simulink model "camara_simul"  (R2018a)
settings: Solver=VariableStepAuto  StartTime=0.0  StopTime=inf  RelTol=1e-3
undefined symbols (not defined in the file or in its folder): IsPositionTracked, IsSkeletonTracked, JointDepthIndices, JointImageIndices, JointTrackingState, JointWorldCoordinates, none, PositionDepthIndices, PositionImageIndices, PositionWorldCoordinates, Rec, SDTV, SegmentationData, SkeletonTrackingID, videoinput
libraries: visionsinks x3, visionconversions x2, simulink x2, visionstatistics x1, visiontextngfix x1, imaqlib x1
settings Model: Creator=Luís Miranda  LastModifiedBy=Luís Miranda

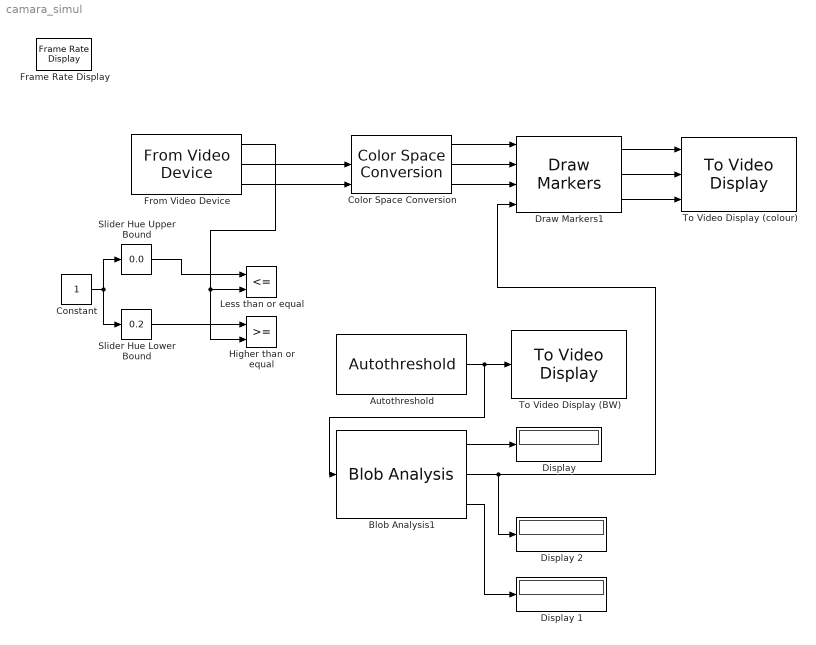
== system camara_simul ==
  Autothreshold : visionconversions/Autothreshold  operator=<=  threshOut=off  effMetricOut=off  userDefinedRange=off  umin=0  umax=255  outOfRngOpt=Warn and saturate  scaleThreshold=off  scaleFactor=1  P1Mode=Specify word length  P1WordLength=32  P1FracLength=30  P2Mode=Specify word length  P2WordLength=32  P2FracLength=22  P3Mode=Specify word length  P3WordLength=32  P3FracLength=14  P4Mode=Binary point scaling  P4WordLength=32  P4FracLength=15  Q1Mode=Specify word length  Q1WordLength=32  Q1FracLength=16  EMMode=Specify word length  EMWordLength=16  EMFracLength=14  roundingMode=Floor  overflowMode=off
      settings: SourceProductName=Computer Vision System Toolbox  SourceProductBaseCode=VP
  Blob Analysis1 : visionstatistics/Blob Analysis  Tag=vipblks_row_conv  area=on  centroid=on  bBox=on  majorAxis=off  minorAxis=off  angle=off  eccentricity=off  equivDiameterSq=off  extent=off  perimeter=off  maxBlobs=1  warnIfNumBlobsExceeded=off  isCount=off  useMinArea=on  minArea=900  useMaxArea=on  maxArea=7800  excludeBorderBlob=off  outDT=double  isOutVarDim=off  isFill=off  fillValues=-1  conn=8  isLabel=off  outputMode=Binary point scaling  outputWordLength=32  outputFracLength=16  firstCoeffMode=Binary point scaling  firstCoeffWordLength=16  firstCoeffFracLength=14  secondCoeffMode=Binary point scaling  secondCoeffWordLength=32  secondCoeffFracLength=16  accumMode=Binary point scaling  accumWordLength=32  accumFracLength=0  prodOutputMode=Binary point scaling  prodOutputWordLength=32  prodOutputFracLength=16  roundingMode=Floor  overflowMode=off
      settings: SourceProductName=Computer Vision System Toolbox
  Color Space Conversion : visionconversions/Color Space  Conversion  conversion=Obsolete  conversionActive=Y'CbCr to R'G'B'  wp_str=D65  rec=Rec. 601 (SDTV)  sys=1125/60/2:1  imagePorts=Separate color signals
      settings: SourceProductName=Computer Vision System Toolbox
  Constant : Constant  OutDataTypeStr=single
  "Display " : Display
  Display 1 : Display
  Display 2 : Display
  Draw Markers1 : visiontextngfix/Draw Markers  shape=Circle  size=3  fill=on  fillClrSource=Specify via dialog  display=User-specified value  intensity=200  color=[255 0 0]  opacity=0.6  viewport=Entire image  antialiasing=off  inType=Obsolete  imagePorts=Separate color signals  prodOutputMode=Binary point scaling  prodOutputWordLength=32  prodOutputFracLength=14  memoryMode=Specify word length  memoryWordLength=16  memoryFracLength=14  roundingMode=Floor  overflowMode=off
      settings: SourceProductName=Computer Vision System Toolbox  SourceProductBaseCode=VP
  Frame Rate Display : visionsinks/Frame Rate Display  UpdateRate=3
      settings: SourceProductName=Computer Vision System Toolbox  SourceProductBaseCode=VP
  From Video Device : imaqlib/From Video Device  DeviceMenu=winvideo 1 (USB2.0 UVC HD Webcam)  Device=winvideo 1 (USB2.0 UVC HD Webcam)  ObjConstructor=videoinput('winvideo', 1)  VideoFormatMenu=MJPG_640x480  VideoFormat=MJPG_640x480  VideoSource=input1  ROIPosition=[0 0 480 640]  EnableHWTrigger=off  TriggerConfiguration=none/none  SampleTime=1/30  OutputPortsMode=Separate color signals  DataType=single  CanDoHWTrigger=no  ReturnedColorSpace=rgb  BlockHandle=1940.0005  ROIWidth=640  ROIHeight=480  ROIColumn=0  ROIRow=0  EngXMLPath=C:\Program Files\MATLAB\R2018a\toolbox\imaq\imaq\private  DevXMLPath=C:\ProgramData\MATLAB\SupportPackages\R2018a\toolbox\imaq\supportpackages\genericvideo\adaptor\win64  EngLibPath=C:\Program Files\MATLAB\R2018a\toolbox\imaq\imaqblks\imaqmex\win64  ColorSpace=rgb  BayerSensorAlignment=grbg  AllMetadata=IsPositionTracked;IsSkeletonTracked;JointDepthIndices;JointImageIndices;JointTrackingState;JointWorldCoordinates;PositionDepthIndices;PositionImageIndices;PositionWorldCoordinates;SegmentationData;SkeletonTrackingID
      settings: SourceProductName=Image Acquisition Toolbox
  Higher than or equal : RelationalOperator  OutDataTypeStr=boolean  RndMeth=Nearest
  Less than or equal : RelationalOperator  Operator=<=  OutDataTypeStr=boolean  RndMeth=Nearest
  Slider Hue Lower Bound : simulink/Math Operations/Slider Gain  gain=0.2  low=0  high=1
  Slider Hue Upper Bound : simulink/Math Operations/Slider Gain  gain=0.0  low=0  high=1
  To Video Display (BW) : visionsinks/To Video Display  windowSizeMode=True size (1:1)  openAtMdlStart=on  fullScreen=off  videoWindowX=75  videoWindowY=52  saveWindowSize=off  videoWindowWidth=160  videoWindowHeight=120  inputColorFormat=RGB  inputType=Obsolete  imagePorts=One multidimensional signal  OutputDevice=On-screen video monitor  dataOrg=Column-major  isWindowOpen=on
      settings: SourceProductName=Computer Vision System Toolbox
  To Video Display (colour) : visionsinks/To Video Display  windowSizeMode=True size (1:1)  openAtMdlStart=on  fullScreen=off  videoWindowX=262  videoWindowY=89  saveWindowSize=off  videoWindowWidth=160  videoWindowHeight=120  inputColorFormat=RGB  inputType=Obsolete  imagePorts=Separate color signals  OutputDevice=On-screen video monitor  dataOrg=Column-major  isWindowOpen=on
      settings: SourceProductName=Computer Vision System Toolbox
  wires:
  Color Space Conversion/3 -> Draw Markers1/3
  Draw Markers1/1 -> To Video Display (colour)/1
  Autothreshold/1 -> Blob Analysis1/1, To Video Display (BW)/1
  Color Space Conversion/1 -> Draw Markers1/1
  From Video Device/3 -> Color Space Conversion/3
  Blob Analysis1/1 -> "Display "/1
  Draw Markers1/2 -> To Video Display (colour)/2
  Draw Markers1/3 -> To Video Display (colour)/3
  From Video Device/2 -> Color Space Conversion/2
  Color Space Conversion/2 -> Draw Markers1/2
  Blob Analysis1/2 -> Display 2/1, Draw Markers1/4
  Blob Analysis1/3 -> Display 1/1
  Slider Hue Lower Bound/1 -> Higher than or equal/1
  Slider Hue Upper Bound/1 -> Less than or equal/1
  Constant/1 -> Slider Hue Lower Bound/1, Slider Hue Upper Bound/1
  From Video Device/1 -> Higher than or equal/2, Less than or equal/2
